simulink model "First_Order_and_Second_Order_Systems"  (R2024b)
settings: Solver=VariableStepAuto  StartTime=0.0  StopTime=20  RelTol=1e-3
values from neighbouring files (symbols this model uses):
  K = 1    [First_order_2nd_order_Lab.m]
  T = R*C    (= 0.001)    [First_Order_System_Analysis.m]    (also in First_order_2nd_order_Lab.m = 0.02)
  wn = 3.5    [First_order_2nd_order_Lab.m]
  zeta = 0.25    [First_order_2nd_order_Lab.m]
settings Model: Creator=LEGION  LastModifiedBy=LEGION

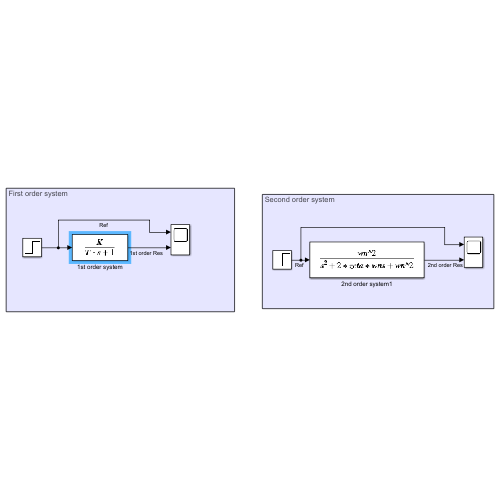
[thumbnail: Simulink's stored preview of the top-level diagram]
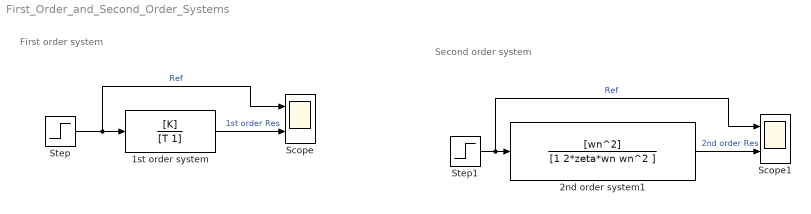
== system First_Order_and_Second_Order_Systems ==
  note: Second order system
  note: First order system
  1st order system : TransferFcn  Numerator=[K]  Denominator=[T 1]
  2nd order system1 : TransferFcn  Numerator=[wn^2]  Denominator=[1 2*zeta*wn wn^2 ]
  Scope : Scope  NumInputPorts=2
  Scope1 : Scope  NumInputPorts=2
  Step : Step  SampleTime=0
  Step1 : Step  SampleTime=0
  wires:
  Step/1 -> Scope/1, 1st order system/1  "Ref"
  1st order system/1 -> Scope/2  "1st order Res"
  Step1/1 -> Scope1/1, 2nd order system1/1  "Ref"
  2nd order system1/1 -> Scope1/2  "2nd order Res"
